simulink model "Querdynamik"  (R2018a)
settings: Solver=ode4  StartTime=0.0  StopTime=10.0  FixedStep=0.001  RelTol=1e-3
model workspace (MAT data in the model file):
  ChStern = 20.803428405
  CvStern = 208.03428405
  deltaControl = 0
  deltaControlled = 1
  deltaH = [1 1 1 1 1 1 1 1 1 1 1 1 1 1 1 1 1 1 1 1 1 1 1 1 1 1 1 1 1 1]
  g = 9.81
  is = 16
  lh = 1.456
  lv = 1.344
  mDivTheta = 0.553571428571
  rSoll = 1
  v = [1 2 3 4 5 6 7 8 9 10 11 12 13 14 15 16 17 18 19 20 21 22 23 24 25 26 27 28 29 30]
values from neighbouring files (symbols this model uses):
  I_s = 16    [untitled.m]
libraries: simulink x1
settings Model: Creator=sebastiankoch  LastModifiedBy=sebastiankoch
settings DebuggingCC: UnderspecifiedInitializationDetection=Classic  MergeDetectMultiDrivingBlocksExec=none

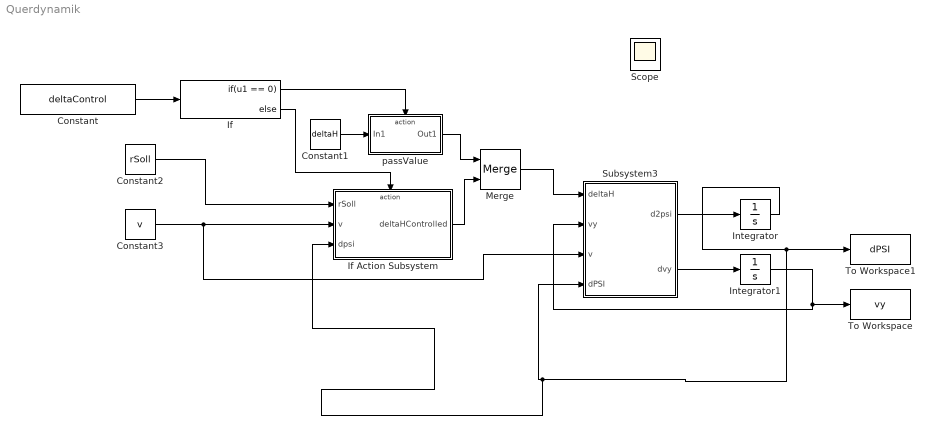
== system Querdynamik ==
  Constant : Constant  Value=deltaControl
  Constant1 : Constant  Value=deltaH
  Constant2 : Constant  Value=rSoll
  Constant3 : Constant  Value=v
  If : If  IfExpression=u1 == 0
  If Action Subsystem : Subsystem  TreatAsAtomicUnit=on
  Integrator : Integrator
  Integrator1 : Integrator
  Merge : Merge  AllowUnequalInputPortWidths=on
  Scope : Scope
  Subsystem3 : Subsystem
  To Workspace : ToWorkspace  VariableName=vy  SampleTime=-1
  To Workspace1 : ToWorkspace  VariableName=dPSI  SampleTime=-1
  passValue : Subsystem  TreatAsAtomicUnit=on
  wires:
  Subsystem3/2(dvy) -> Integrator1/1
  Subsystem3/1("d2psi ") -> Integrator/1
  Integrator1/1 -> Subsystem3/2(vy), To Workspace/1
  Constant/1 -> If/1
  If/1 -> passValue/Action
  Constant1/1 -> passValue/1(In1)
  If/2 -> If Action Subsystem/Action
  Constant2/1 -> If Action Subsystem/1(rSoll)
  Constant3/1 -> Subsystem3/3(v), If Action Subsystem/2(v)
  passValue/1(Out1) -> Merge/1
  If Action Subsystem/1(deltaHControlled) -> Merge/2
  Merge/1 -> Subsystem3/1(deltaH)
  Integrator/1 -> If Action Subsystem/3(dpsi), Subsystem3/4(dPSI), To Workspace1/1

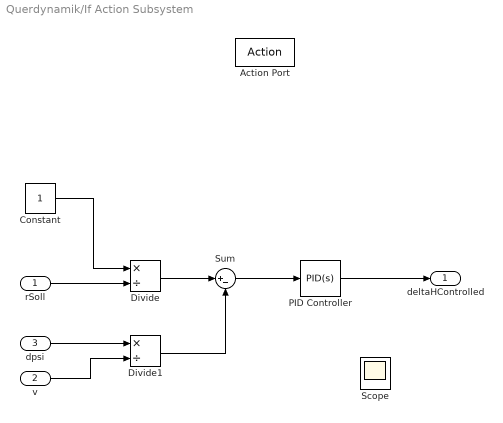
== system Querdynamik/If Action Subsystem ==
  rSoll : Inport
  v : Inport  Port=2
  dpsi : Inport  Port=3
  Action Port : ActionPort  ActionType=else
  Constant : Constant
  Divide : Product  Inputs=*/
  Divide1 : Product  Inputs=*/
  PID Controller : simulink/Continuous/PID Controller  Controller=PID  TimeDomain=Continuous-time  SampleTime=-1  IntegratorMethod=Forward Euler  FilterMethod=Forward Euler  Form=Parallel  UseFilter=on  ControllerParametersSource=internal  P=504.712447211076  I=1502.6695131007  D=0  N=100  InitialConditionSource=internal  InitialConditionForIntegrator=0  InitialConditionForFilter=0  ExternalReset=none  LimitOutput=off  UpperSaturationLimit=inf  LowerSaturationLimit=-inf  LinearizeAsGain=on  AntiWindupMode=none  Kb=1  TrackingMode=off  Kt=1  PParamMin=[]  PParamMax=[]  IParamMin=[]  IParamMax=[]  DParamMin=[]  DParamMax=[]  NParamMin=[]  NParamMax=[]  KbParamMin=[]  KbParamMax=[]  KtParamMin=[]  KtParamMax=[]  POutMin=[]  POutMax=[]  IOutMin=[]  IOutMax=[]  DOutMin=[]  DOutMax=[]  NOutMin=[]  NOutMax=[]  KbOutMin=[]  KbOutMax=[]  KtOutMin=[]  KtOutMax=[]  IntegratorOutMin=[]  IntegratorOutMax=[]  FilterOutMin=[]  FilterOutMax=[]  SumOutMin=[]  SumOutMax=[]  SumI1OutMin=[]  SumI1OutMax=[]  SumI2OutMin=[]  SumI2OutMax=[]  SumI3OutMin=[]  SumI3OutMax=[]  SumDOutMin=[]  SumDOutMax=[]  SaturationOutMin=[]  SaturationOutMax=[]  IntegratorContinuousStateAttributes=''  IntegratorStateMustResolveToSignalObject=off  IntegratorRTWStateStorageClass=Auto  FilterContinuousStateAttributes=''  FilterStateMustResolveToSignalObject=off  FilterRTWStateStorageClass=Auto  DifferentiatorICPrevScaledInput=0  DifferentiatorOutMin=[]  DifferentiatorOutMax=[]  FilterDiffOutCoefMin=[]  FilterDiffOutCoefMax=[]  SumDenOutMin=[]  SumDenOutMax=[]  SumNumOutMin=[]  SumNumOutMax=[]  ReciprocalOutMin=[]  ReciprocalOutMax=[]  DivideOutMin=[]  DivideOutMax=[]  TunerSelectOption=Transfer Function Based (PID Tuner App)
  Scope : Scope
  Sum : Sum  Inputs=|+-
  deltaHControlled : Outport
  wires:
  Constant/1 -> Divide/1
  rSoll/1 -> Divide/2
  Divide/1 -> Sum/1
  dpsi/1 -> Divide1/1
  v/1 -> Divide1/2
  Divide1/1 -> Sum/2
  Sum/1 -> PID Controller/1
  PID Controller/1 -> deltaHControlled/1

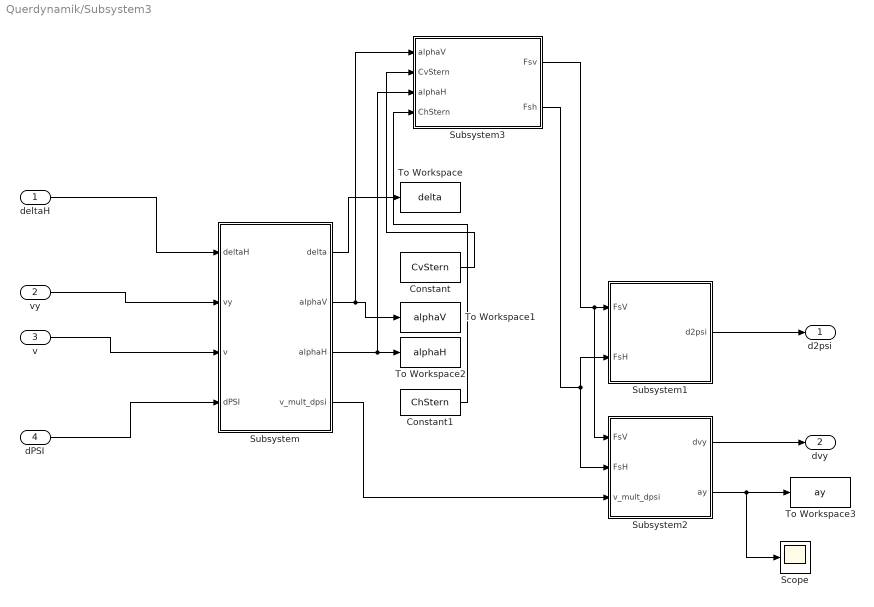
== system Querdynamik/Subsystem3 ==
  deltaH : Inport
  vy : Inport  Port=2
  v : Inport  Port=3
  dPSI : Inport  Port=4
  Constant : Constant  Value=CvStern
  Constant1 : Constant  Value=ChStern
  Scope : Scope
  Subsystem : Subsystem
  Subsystem1 : Subsystem
  Subsystem2 : Subsystem
  Subsystem3 : Subsystem
  To Workspace : ToWorkspace  VariableName=delta  SampleTime=-1
  To Workspace1 : ToWorkspace  VariableName=alphaV  SampleTime=-1
  To Workspace2 : ToWorkspace  VariableName=alphaH  SampleTime=-1
  To Workspace3 : ToWorkspace  VariableName=ay  SampleTime=-1
  "d2psi " : Outport
  dvy : Outport  Port=2
  wires:
  v/1 -> Subsystem/3(v)
  Subsystem/4(v_mult_dpsi) -> Subsystem2/3("v_mult_dpsi ")
  Subsystem2/1(dvy) -> dvy/1
  dPSI/1 -> Subsystem/4(dPSI)
  Subsystem/1(delta) -> To Workspace/1
  Subsystem3/2(Fsh) -> Subsystem1/2(FsH), Subsystem2/2(FsH)
  Subsystem1/1(d2psi) -> "d2psi "/1
  vy/1 -> Subsystem/2(vy)
  Subsystem/3(alphaH) -> Subsystem3/3(alphaH), To Workspace2/1
  Subsystem/2(alphaV) -> Subsystem3/1(alphaV), To Workspace1/1
  Subsystem2/2(ay) -> Scope/1, To Workspace3/1
  deltaH/1 -> Subsystem/1(deltaH)
  Subsystem3/1(Fsv) -> Subsystem2/1(FsV), Subsystem1/1(FsV)
  Constant/1 -> Subsystem3/2(CvStern)
  Constant1/1 -> Subsystem3/4(ChStern)

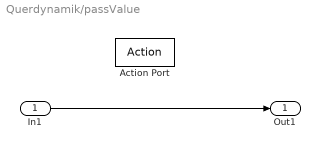
== system Querdynamik/passValue ==
  In1 : Inport
  Action Port : ActionPort  ActionType=then
  Out1 : Outport
  wires:
  In1/1 -> Out1/1

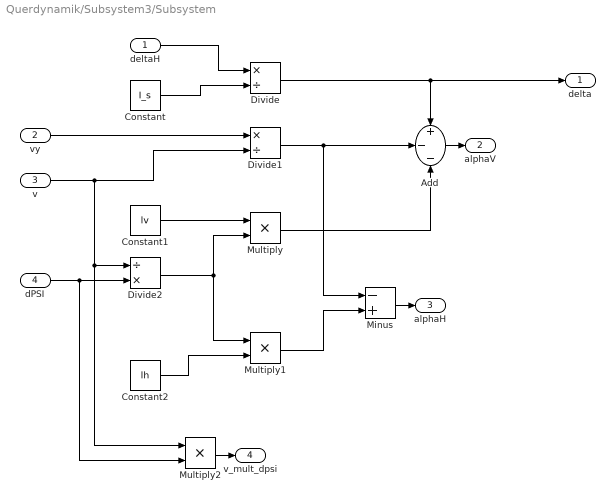
== system Querdynamik/Subsystem3/Subsystem ==
  deltaH : Inport
  vy : Inport  Port=2
  v : Inport  Port=3
  dPSI : Inport  Port=4
  Add : Sum  Inputs=+--
  Constant : Constant  Value=I_s
  Constant1 : Constant  Value=lv
  Constant2 : Constant  Value=lh
  Divide : Product  Inputs=*/
  Divide1 : Product  Inputs=*/
  Divide2 : Product  Inputs=/*
  Minus : Sum  Inputs=-+
  Multiply : Product
  Multiply1 : Product
  Multiply2 : Product
  delta : Outport
  alphaV : Outport  Port=2
  alphaH : Outport  Port=3
  v_mult_dpsi : Outport  Port=4
  wires:
  deltaH/1 -> Divide/1
  Add/1 -> alphaV/1
  dPSI/1 -> Multiply2/2, Divide2/2
  Multiply1/1 -> Minus/2
  v/1 -> Multiply2/1, Divide2/1, Divide1/2
  Divide/1 -> delta/1, Add/1
  Constant/1 -> Divide/2
  Multiply2/1 -> v_mult_dpsi/1
  Constant2/1 -> Multiply1/2
  Minus/1 -> alphaH/1
  Multiply/1 -> Add/3
  Constant1/1 -> Multiply/1
  vy/1 -> Divide1/1
  Divide2/1 -> Multiply1/1, Multiply/2
  Divide1/1 -> Add/2, Minus/1

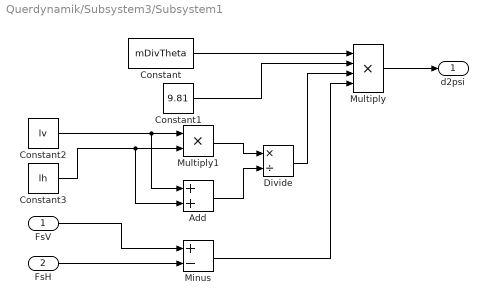
== system Querdynamik/Subsystem3/Subsystem1 ==
  FsV : Inport
  FsH : Inport  Port=2
  Add : Sum
  Constant : Constant  Value=mDivTheta
  Constant1 : Constant  Value=9.81
  Constant2 : Constant  Value=lv
  Constant3 : Constant  Value=lh
  Divide : Product  Inputs=*/
  Minus : Sum  Inputs=+-
  Multiply : Product  Inputs=4
  Multiply1 : Product
  d2psi : Outport
  wires:
  Constant/1 -> Multiply/1
  Constant1/1 -> Multiply/2
  Constant2/1 -> Add/1, Multiply1/1
  Constant3/1 -> Add/2, Multiply1/2
  Multiply1/1 -> Divide/1
  Add/1 -> Divide/2
  Divide/1 -> Multiply/3
  Multiply/1 -> d2psi/1
  Minus/1 -> Multiply/4
  FsH/1 -> Minus/2
  FsV/1 -> Minus/1

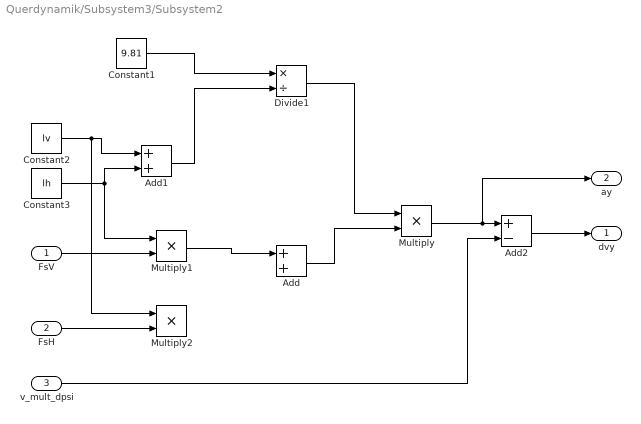
== system Querdynamik/Subsystem3/Subsystem2 ==
  FsV : Inport
  FsH : Inport  Port=2
  "v_mult_dpsi " : Inport  Port=3
  Add : Sum
  Add1 : Sum
  Add2 : Sum  Inputs=+-
  Constant1 : Constant  Value=9.81
  Constant2 : Constant  Value=lv
  Constant3 : Constant  Value=lh
  Divide1 : Product  Inputs=*/
  Multiply : Product
  Multiply1 : Product
  Multiply2 : Product
  dvy : Outport
  ay : Outport  Port=2
  wires:
  Constant2/1 -> Multiply2/1, Add1/1
  Constant3/1 -> Multiply1/1, Add1/2
  Add1/1 -> Divide1/2
  Constant1/1 -> Divide1/1
  Divide1/1 -> Multiply/1
  Add/1 -> Multiply/2
  FsV/1 -> Multiply1/2
  Multiply1/1 -> Add/1
  FsH/1 -> Multiply2/2
  Multiply/1 -> ay/1, Add2/1
  "v_mult_dpsi "/1 -> Add2/2
  Add2/1 -> dvy/1

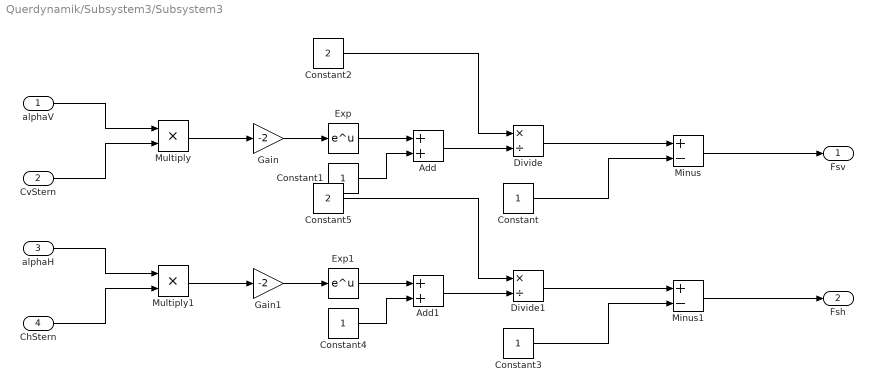
== system Querdynamik/Subsystem3/Subsystem3 ==
  alphaV : Inport
  CvStern : Inport  Port=2
  alphaH : Inport  Port=3
  ChStern : Inport  Port=4
  Add : Sum
  Add1 : Sum
  Constant{,1,3..4} (4 alike) : Constant
  Constant2 : Constant  Value=2
  Constant5 : Constant  Value=2
  Divide : Product  Inputs=*/
  Divide1 : Product  Inputs=*/
  Exp : Math  SaturateOnIntegerOverflow=on
  Exp1 : Math  SaturateOnIntegerOverflow=on
  Gain : Gain  Gain=-2
  Gain1 : Gain  Gain=-2
  Minus : Sum  Inputs=+-
  Minus1 : Sum  Inputs=+-
  Multiply : Product
  Multiply1 : Product
  Fsv : Outport
  Fsh : Outport  Port=2
  wires:
  Multiply/1 -> Gain/1
  Gain/1 -> Exp/1
  alphaV/1 -> Multiply/1
  CvStern/1 -> Multiply/2
  Exp/1 -> Add/1
  Constant1/1 -> Add/2
  Add/1 -> Divide/2
  Constant2/1 -> Divide/1
  Constant/1 -> Minus/2
  Divide/1 -> Minus/1
  Minus/1 -> Fsv/1
  ChStern/1 -> Multiply1/2
  Exp1/1 -> Add1/1
  Divide1/1 -> Minus1/1
  Constant4/1 -> Add1/2
  Minus1/1 -> Fsh/1
  Add1/1 -> Divide1/2
  Multiply1/1 -> Gain1/1
  Gain1/1 -> Exp1/1
  Constant3/1 -> Minus1/2
  alphaH/1 -> Multiply1/1
  Constant5/1 -> Divide1/1
